simulink model "findPosition_th"  (R2018b)
settings: Solver=VariableStepAuto  StartTime=0.0  StopTime=10.0  RelTol=1e-3
undefined symbols (not defined in the file or in its folder): getVal, GFC2Bottom, GFC2Side, GFC2Slant
libraries: findPosition_ul x1
settings Model: Creator=mae-ncsucore  LastModifiedBy=MAE-NCSUCORE

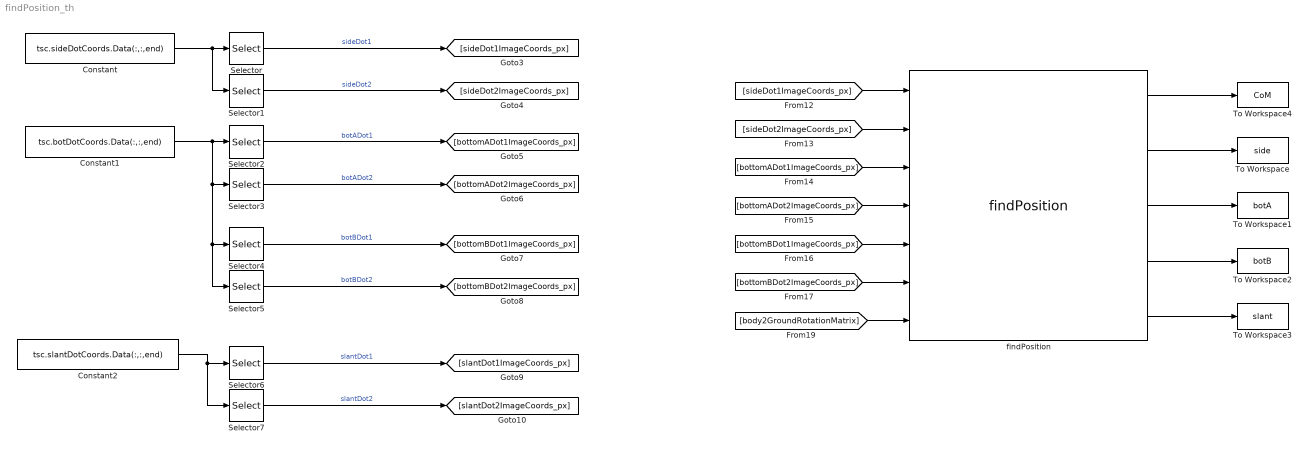
== system findPosition_th ==
  Constant : Constant  Value=tsc.sideDotCoords.Data(:,:,end)
  Constant1 : Constant  Value=tsc.botDotCoords.Data(:,:,end)
  Constant2 : Constant  Value=tsc.slantDotCoords.Data(:,:,end)
  Selector : Selector  InputPortWidth=4  IndexOptions=Index vector (dialog)  Indices=[1 2]  OutputSizes=1
  Selector1 : Selector  InputPortWidth=4  IndexOptions=Index vector (dialog)  Indices=[3 4]  OutputSizes=1
  Selector2 : Selector  InputPortWidth=8  IndexOptions=Index vector (dialog)  Indices=[1 2]  OutputSizes=1
  Selector3 : Selector  InputPortWidth=8  IndexOptions=Index vector (dialog)  Indices=[3 4]  OutputSizes=1
  Selector4 : Selector  InputPortWidth=8  IndexOptions=Index vector (dialog)  Indices=[5 6]  OutputSizes=1
  Selector5 : Selector  InputPortWidth=8  IndexOptions=Index vector (dialog)  Indices=[7 8]  OutputSizes=1
  Selector6 : Selector  InputPortWidth=4  IndexOptions=Index vector (dialog)  Indices=[1 2]  OutputSizes=1
  Selector7 : Selector  InputPortWidth=4  IndexOptions=Index vector (dialog)  Indices=[3 4]  OutputSizes=1
  To Workspace : ToWorkspace  VariableName=side  SaveFormat=Timeseries  SampleTime=-1
  To Workspace1 : ToWorkspace  VariableName=botA  SaveFormat=Timeseries  SampleTime=-1
  To Workspace2 : ToWorkspace  VariableName=botB  SaveFormat=Timeseries  SampleTime=-1
  To Workspace3 : ToWorkspace  VariableName=slant  SaveFormat=Timeseries  SampleTime=-1
  To Workspace4 : ToWorkspace  VariableName=CoM  SaveFormat=Timeseries  SampleTime=-1
  findPosition : findPosition_ul/findPosition  sideCameraPositionVec_cm=getVal('sideCamPosVec_cm')  bottomCameraPositionVec_cm=getVal('botCamPosVec_cm')  slantCameraPositionVec_cm=getVal('slntCamPosVec_cm')  sideDotPositionVec_cm=getVal('sideDotSepDist_cm')  bottomDotAPositionVec_cm=getVal('botADotSepDist_cm')  bottomDotBPositionVec_cm=getVal('botBDotSepDist_cm')  side2GroundRotationMatrix=GFC2Side'  bot2GroundRotationMatrix=GFC2Bottom'  slant2GroundRotationMatrix=GFC2Slant'  initialCoMPositionVec_cm=getVal('initCoMPosVec_cm')  imageDims=getVal('sideImageSize_px')  cameraFOVAngle_deg=getVal('cameraFOV_deg')
  wires:
  findPosition/2 -> To Workspace/1
  findPosition/5 -> To Workspace3/1
  findPosition/4 -> To Workspace2/1
  findPosition/3 -> To Workspace1/1
  findPosition/1 -> To Workspace4/1
  Selector6/1 -> [slantDot1ImageCoords_px]  "slantDot1"
  Selector4/1 -> [bottomBDot1ImageCoords_px]  "botBDot1"
  Constant2/1 -> Selector7/1, Selector6/1
  Selector7/1 -> [slantDot2ImageCoords_px]  "slantDot2"
  Selector3/1 -> [bottomADot2ImageCoords_px]  "botADot2"
  Selector1/1 -> [sideDot2ImageCoords_px]  "sideDot2"
  Selector5/1 -> [bottomBDot2ImageCoords_px]  "botBDot2"
  Constant/1 -> Selector/1, Selector1/1
  Selector/1 -> [sideDot1ImageCoords_px]  "sideDot1"
  Selector2/1 -> [bottomADot1ImageCoords_px]  "botADot1"
  [bottomADot2ImageCoords_px] -> findPosition/4
  [bottomBDot2ImageCoords_px] -> findPosition/6
  [bottomBDot1ImageCoords_px] -> findPosition/5
  [body2GroundRotationMatrix] -> findPosition/7
  [sideDot1ImageCoords_px] -> findPosition/1
  [bottomADot1ImageCoords_px] -> findPosition/3
  [sideDot2ImageCoords_px] -> findPosition/2
  Constant1/1 -> Selector2/1, Selector5/1, Selector4/1, Selector3/1
